simulink model "vco"  (R2019b)
settings: Solver=ode113  StartTime=0.0  StopTime=1e-6  RelTol=1e-3
values from neighbouring files (symbols this model uses):
  fs = fB*2    (= 10000000)    [vco_counter_m.m]    (also in vco_m.m = 1600000000)
  fvco = 1000e6    (= 1000000000)    [vco_counter_m.m]    (also in vco_m.m = 1600000000)
  ts = 1/fs    (= 1e-07)    [vco_counter_m.m]    (also in vco_m.m = 6.25e-10)
  tsys_res = 1e-11    [vco_counter_m.m]    (also in vco_m.m = 6.25e-10)
  tvco = 1/fvco    (= 6.25e-10)    [vco_m.m]
  vco_inverter_nums = 33    [vco_m.m]
libraries: simulink_extras x66
(part 1 of 2)
settings Model: Creator=benve  LastModifiedBy=benve

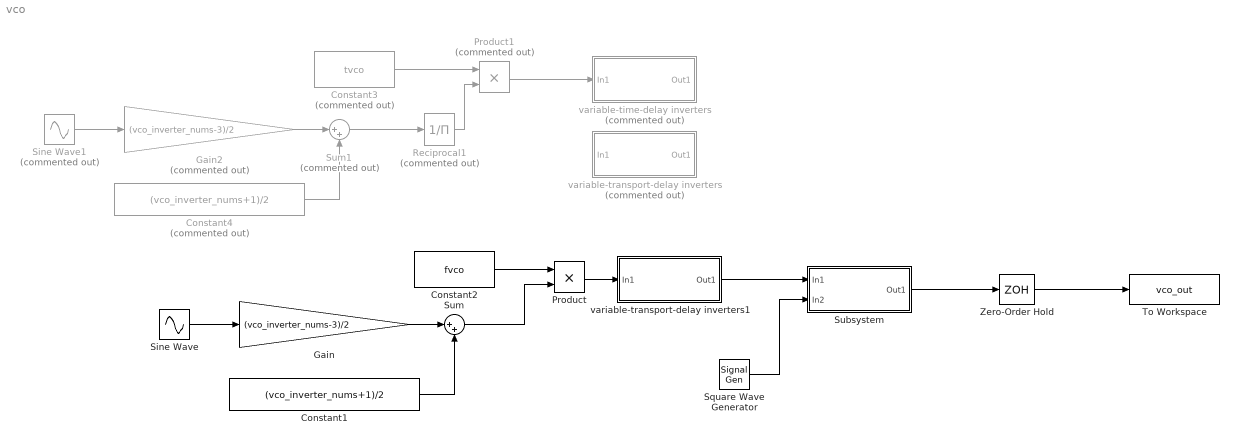
== system vco ==
  Constant1 : Constant  Value=(vco_inverter_nums+1)/2  SampleTime=tsys_res
  Constant2 : Constant  Value=fvco  SampleTime=tsys_res
  Constant3 : Constant  Commented=on  Value=tvco  SampleTime=tsys_res
  Constant4 : Constant  Commented=on  Value=(vco_inverter_nums+1)/2  SampleTime=tsys_res
  Gain : Gain  Gain=(vco_inverter_nums-3)/2
  Gain2 : Gain  Commented=on  Gain=(vco_inverter_nums-3)/2
  Product : Product
  Product1 : Product  Commented=on
  Reciprocal1 : Product  Commented=on  Inputs=/
  Sine Wave : Sin  Frequency=13e6*2*pi  SampleTime=ts
  Sine Wave1 : Sin  Commented=on  Frequency=13e6*2*pi  SampleTime=ts
  Square Wave Generator : SignalGenerator  WaveForm=square  Frequency=fs
  Subsystem : Subsystem
  Sum : Sum  Inputs=|++
  Sum1 : Sum  Commented=on  Inputs=|++
  To Workspace : ToWorkspace  VariableName=vco_out  SampleTime=-1
      settings: Save2DSignal=2-D array (concatenate along first dimension)
  Zero-Order Hold : ZeroOrderHold  SampleTime=ts
  variable-time-delay inverters : Subsystem  Commented=on  TreatAsAtomicUnit=on
      settings: RTWFcnNameOpts=Use subsystem name  RTWFileNameOpts=Use function name
  variable-transport-delay inverters : Subsystem  Commented=on  TreatAsAtomicUnit=on
      settings: RTWFcnNameOpts=Use subsystem name  RTWFileNameOpts=Use function name
  variable-transport-delay inverters1 : Subsystem  TreatAsAtomicUnit=on
      settings: RTWFcnNameOpts=Use subsystem name  RTWFileNameOpts=Use function name
  wires:
  Square Wave Generator/1 -> Subsystem/2(In2)
  Subsystem/1(Out1) -> Zero-Order Hold/1
  Zero-Order Hold/1 -> To Workspace/1
  variable-transport-delay inverters1/1(Out1) -> Subsystem/1(In1)
  Product/1 -> variable-transport-delay inverters1/1(In1)
  Reciprocal1/1 -> Product1/2
  Sine Wave1/1 -> Gain2/1
  Gain2/1 -> Sum1/1
  Constant3/1 -> Product1/1
  Constant4/1 -> Sum1/2
  Sum1/1 -> Reciprocal1/1
  Product1/1 -> variable-time-delay inverters/1(In1)
  Constant2/1 -> Product/1
  Sine Wave/1 -> Gain/1
  Gain/1 -> Sum/1
  Constant1/1 -> Sum/2
  Sum/1 -> Product/2

== system vco/Subsystem ==
  In1 : Inport
  In2 : Inport  Port=2
  "10 XORs " : Subsystem
  10 XORs 1 : Subsystem
  10 XORs 2 : Subsystem
  3 XORs : Subsystem
  Adder : Subsystem
  Bus Selector : BusSelector  OutputSignals=signal1,signal2,signal3,signal4
  stage1 - 10registers : Subsystem
  stage1 - 10registers1 : Subsystem
  stage1 - 10registers2 : Subsystem
  stage1 - 3registers : Subsystem
  stage2 - 10registers1 : Subsystem
  stage2 - 10registers2 : Subsystem
  stage2 - 10registers3 : Subsystem
  stage2 - 3registers : Subsystem
  Out1 : Outport
  wires:
  "10 XORs "/1(Out2) -> Adder/1(In1)
  stage2 - 10registers3/1(Out1) -> "10 XORs "/2(In3)
  Adder/1(Out1) -> Out1/1
  Bus Selector/4 -> stage1 - 3registers/1(In1)  "<signal4>"
  stage2 - 10registers1/1(Out1) -> 10 XORs 1/2(In3)
  stage2 - 10registers2/1(Out1) -> 10 XORs 2/2(In3)
  10 XORs 1/1(Out2) -> Adder/2(In2)
  Bus Selector/3 -> stage1 - 10registers2/1(In1)  "<signal3>"
  stage1 - 10registers1/1(Out1) -> 10 XORs 1/1(In2), stage2 - 10registers1/1(In1)
  10 XORs 2/1(Out2) -> Adder/3(In3)
  stage1 - 3registers/1(Out1) -> 3 XORs/1(In1), stage2 - 3registers/1(In1)
  In2/1 -> stage2 - 3registers/2(In2), stage2 - 10registers3/2(In2), stage2 - 10registers1/2(In2), stage2 - 10registers2/2(In2), stage1 - 3registers/2(In2), stage1 - 10registers2/2(In2), stage1 - 10registers/2(In2), stage1 - 10registers1/2(In2)  "SAMP_CLK"
  In1/1 -> Bus Selector/1
  stage1 - 10registers2/1(Out1) -> 10 XORs 2/1(In2), stage2 - 10registers2/1(In1)
  3 XORs/1(Out1) -> Adder/4(In4)
  stage2 - 3registers/1(Out1) -> 3 XORs/2(In2)
  Bus Selector/2 -> stage1 - 10registers1/1(In1)  "<signal2>"
  stage1 - 10registers/1(Out1) -> "10 XORs "/1(In2), stage2 - 10registers3/1(In1)
  Bus Selector/1 -> stage1 - 10registers/1(In1)  "<signal1>"

== system vco/variable-time-delay inverters ==
  In1 : Inport
  " 3 inverters" : Subsystem
  10 inverters : Subsystem
  10 inverters1 : Subsystem
  10 inverters2 : Subsystem
  Bus Creator : BusCreator  Inputs=4
  Out1 : Outport
  wires:
  Bus Creator/1 -> Out1/1
  10 inverters/1(Out2) -> 10 inverters1/1(In1)
  10 inverters1/1(Out2) -> 10 inverters2/1(In1)
  10 inverters2/1(Out2) -> " 3 inverters"/1(In1)
  10 inverters/2(Out1) -> Bus Creator/1
  10 inverters1/2(Out1) -> Bus Creator/2
  10 inverters2/2(Out1) -> Bus Creator/3
  " 3 inverters"/1(Out2) -> 10 inverters/1(In1)
  In1/1 -> 10 inverters1/2(In2), 10 inverters2/2(In2), " 3 inverters"/2(In2), 10 inverters/2(In2)  "delay"
  " 3 inverters"/2(Out1) -> Bus Creator/4

== system vco/variable-transport-delay inverters ==
  In1 : Inport
  " 3 inverters" : Subsystem
  10 inverters : Subsystem
  10 inverters1 : Subsystem
  10 inverters2 : Subsystem
  Bus Creator : BusCreator  Inputs=4
  Out1 : Outport
  wires:
  Bus Creator/1 -> Out1/1
  10 inverters/1(Out2) -> 10 inverters1/1(In1)
  10 inverters1/1(Out2) -> 10 inverters2/1(In1)
  10 inverters2/1(Out2) -> " 3 inverters"/1(In1)
  10 inverters/2(Out1) -> Bus Creator/1
  10 inverters1/2(Out1) -> Bus Creator/2
  10 inverters2/2(Out1) -> Bus Creator/3
  " 3 inverters"/1(Out2) -> 10 inverters/1(In1)
  In1/1 -> 10 inverters1/2(In2), 10 inverters2/2(In2), " 3 inverters"/2(In2), 10 inverters/2(In2)  "delay"
  " 3 inverters"/2(Out1) -> Bus Creator/4

== system vco/variable-transport-delay inverters1 ==
  In1 : Inport
  10 inverters : Subsystem
  10 inverters1 : Subsystem
  10 inverters2 : Subsystem
  3 inverters : Subsystem
  Bus Creator : BusCreator  Inputs=4
  Out1 : Outport
  wires:
  Bus Creator/1 -> Out1/1
  10 inverters1/1(Out2) -> 10 inverters2/1(In1)
  10 inverters2/1(Out2) -> 3 inverters/1(In1)
  10 inverters1/2(Out1) -> Bus Creator/2
  10 inverters2/2(Out1) -> Bus Creator/3
  In1/1 -> 10 inverters/2(In2), 10 inverters1/2(In2), 10 inverters2/2(In2), 3 inverters/2(In2)  "delay"
  10 inverters/1(Out2) -> 10 inverters1/1(In1)
  10 inverters/2(Out1) -> Bus Creator/1
  3 inverters/1(Out2) -> 10 inverters/1(In1)
  3 inverters/2(Out1) -> Bus Creator/4

== system vco/Subsystem/10 XORs  ==
  In2 : Inport
  In3 : Inport  Port=2
  Bus Creator : BusCreator  Inputs=2
  Bus Creator1 : BusCreator  Inputs=10
  Bus Selector2 : BusSelector  OutputSignals=signal1.signal1,signal2.signal1,signal1.signal2,signal2.signal2,signal1.signal3,signal2.signal3,signal1.signal4,signal2.signal4,signal1.signal5,signal2.signal5,signal1.signal6,signal2.signal6,signal1.signal7,signal2.signal7,signal1.signal8,signal2.signal8,signal1.signal9,signal2.signal9,signal1.signal10,signal2.signal10
  XOR{,1..9} (10 alike) : Logic  Operator=XOR  IconShape=distinctive  AllPortsSameDT=off  OutDataTypeStr=boolean
  Out2 : Outport
  wires:
  XOR2/1 -> Bus Creator1/3
  XOR/1 -> Bus Creator1/1
  Bus Selector2/19 -> XOR9/1  "<signal10>"
  XOR7/1 -> Bus Creator1/8
  Bus Selector2/13 -> XOR6/1  "<signal7>"
  XOR8/1 -> Bus Creator1/9
  XOR9/1 -> Bus Creator1/10
  Bus Selector2/16 -> XOR7/2  "<signal8>"
  Bus Selector2/5 -> XOR2/1  "<signal3>"
  Bus Selector2/17 -> XOR8/1  "<signal9>"
  Bus Creator1/1 -> Out2/1
  Bus Selector2/9 -> XOR4/1  "<signal5>"
  XOR5/1 -> Bus Creator1/6
  XOR6/1 -> Bus Creator1/7
  Bus Selector2/18 -> XOR8/2  "<signal9>"
  XOR1/1 -> Bus Creator1/2
  Bus Selector2/12 -> XOR5/2  "<signal6>"
  Bus Selector2/3 -> XOR1/1  "<signal2>"
  Bus Selector2/4 -> XOR1/2  "<signal2>"
  Bus Selector2/15 -> XOR7/1  "<signal8>"
  Bus Selector2/11 -> XOR5/1  "<signal6>"
  In3/1 -> Bus Creator/2
  Bus Selector2/8 -> XOR3/2  "<signal4>"
  Bus Selector2/6 -> XOR2/2  "<signal3>"
  Bus Selector2/14 -> XOR6/2  "<signal7>"
  Bus Creator/1 -> Bus Selector2/1
  XOR4/1 -> Bus Creator1/5
  Bus Selector2/2 -> XOR/2  "<signal1>"
  Bus Selector2/10 -> XOR4/2  "<signal5>"
  Bus Selector2/7 -> XOR3/1  "<signal4>"
  Bus Selector2/1 -> XOR/1  "<signal1>"
  Bus Selector2/20 -> XOR9/2  "<signal10>"
  In2/1 -> Bus Creator/1
  XOR3/1 -> Bus Creator1/4

== system vco/Subsystem/10 XORs 1 ==
  In2 : Inport
  In3 : Inport  Port=2
  Bus Creator : BusCreator  Inputs=2
  Bus Creator1 : BusCreator  Inputs=10
  Bus Selector2 : BusSelector  OutputSignals=signal1.signal1,signal2.signal1,signal1.signal2,signal2.signal2,signal1.signal3,signal2.signal3,signal1.signal4,signal2.signal4,signal1.signal5,signal2.signal5,signal1.signal6,signal2.signal6,signal1.signal7,signal2.signal7,signal1.signal8,signal2.signal8,signal1.signal9,signal2.signal9,signal1.signal10,signal2.signal10
  XOR{,1..9} (10 alike) : Logic  Operator=XOR  IconShape=distinctive  AllPortsSameDT=off  OutDataTypeStr=boolean
  Out2 : Outport
  wires:
  XOR2/1 -> Bus Creator1/3
  XOR/1 -> Bus Creator1/1
  Bus Selector2/19 -> XOR9/1  "<signal10>"
  XOR7/1 -> Bus Creator1/8
  Bus Selector2/13 -> XOR6/1  "<signal7>"
  XOR8/1 -> Bus Creator1/9
  XOR9/1 -> Bus Creator1/10
  Bus Selector2/16 -> XOR7/2  "<signal8>"
  Bus Selector2/5 -> XOR2/1  "<signal3>"
  Bus Selector2/17 -> XOR8/1  "<signal9>"
  Bus Creator1/1 -> Out2/1
  Bus Selector2/9 -> XOR4/1  "<signal5>"
  XOR5/1 -> Bus Creator1/6
  XOR6/1 -> Bus Creator1/7
  Bus Selector2/18 -> XOR8/2  "<signal9>"
  XOR1/1 -> Bus Creator1/2
  Bus Selector2/12 -> XOR5/2  "<signal6>"
  Bus Selector2/3 -> XOR1/1  "<signal2>"
  Bus Selector2/4 -> XOR1/2  "<signal2>"
  Bus Selector2/15 -> XOR7/1  "<signal8>"
  Bus Selector2/11 -> XOR5/1  "<signal6>"
  In3/1 -> Bus Creator/2
  Bus Selector2/8 -> XOR3/2  "<signal4>"
  Bus Selector2/6 -> XOR2/2  "<signal3>"
  Bus Selector2/14 -> XOR6/2  "<signal7>"
  Bus Creator/1 -> Bus Selector2/1
  XOR4/1 -> Bus Creator1/5
  Bus Selector2/2 -> XOR/2  "<signal1>"
  Bus Selector2/10 -> XOR4/2  "<signal5>"
  Bus Selector2/7 -> XOR3/1  "<signal4>"
  Bus Selector2/1 -> XOR/1  "<signal1>"
  Bus Selector2/20 -> XOR9/2  "<signal10>"
  In2/1 -> Bus Creator/1
  XOR3/1 -> Bus Creator1/4

== system vco/Subsystem/10 XORs 2 ==
  In2 : Inport
  In3 : Inport  Port=2
  Bus Creator : BusCreator  Inputs=2
  Bus Creator1 : BusCreator  Inputs=10
  Bus Selector2 : BusSelector  OutputSignals=signal1.signal1,signal2.signal1,signal1.signal2,signal2.signal2,signal1.signal3,signal2.signal3,signal1.signal4,signal2.signal4,signal1.signal5,signal2.signal5,signal1.signal6,signal2.signal6,signal1.signal7,signal2.signal7,signal1.signal8,signal2.signal8,signal1.signal9,signal2.signal9,signal1.signal10,signal2.signal10
  XOR{,1..9} (10 alike) : Logic  Operator=XOR  IconShape=distinctive  AllPortsSameDT=off  OutDataTypeStr=boolean
  Out2 : Outport
  wires:
  XOR2/1 -> Bus Creator1/3
  XOR/1 -> Bus Creator1/1
  Bus Selector2/19 -> XOR9/1  "<signal10>"
  XOR7/1 -> Bus Creator1/8
  Bus Selector2/13 -> XOR6/1  "<signal7>"
  XOR8/1 -> Bus Creator1/9
  XOR9/1 -> Bus Creator1/10
  Bus Selector2/16 -> XOR7/2  "<signal8>"
  Bus Selector2/5 -> XOR2/1  "<signal3>"
  Bus Selector2/17 -> XOR8/1  "<signal9>"
  Bus Creator1/1 -> Out2/1
  Bus Selector2/9 -> XOR4/1  "<signal5>"
  XOR5/1 -> Bus Creator1/6
  XOR6/1 -> Bus Creator1/7
  Bus Selector2/18 -> XOR8/2  "<signal9>"
  XOR1/1 -> Bus Creator1/2
  Bus Selector2/12 -> XOR5/2  "<signal6>"
  Bus Selector2/3 -> XOR1/1  "<signal2>"
  Bus Selector2/4 -> XOR1/2  "<signal2>"
  Bus Selector2/15 -> XOR7/1  "<signal8>"
  Bus Selector2/11 -> XOR5/1  "<signal6>"
  In3/1 -> Bus Creator/2
  Bus Selector2/8 -> XOR3/2  "<signal4>"
  Bus Selector2/6 -> XOR2/2  "<signal3>"
  Bus Selector2/14 -> XOR6/2  "<signal7>"
  Bus Creator/1 -> Bus Selector2/1
  XOR4/1 -> Bus Creator1/5
  Bus Selector2/2 -> XOR/2  "<signal1>"
  Bus Selector2/10 -> XOR4/2  "<signal5>"
  Bus Selector2/7 -> XOR3/1  "<signal4>"
  Bus Selector2/1 -> XOR/1  "<signal1>"
  Bus Selector2/20 -> XOR9/2  "<signal10>"
  In2/1 -> Bus Creator/1
  XOR3/1 -> Bus Creator1/4

== system vco/Subsystem/3 XORs ==
  In1 : Inport
  In2 : Inport  Port=2
  Bus Creator : BusCreator  Inputs=2
  Bus Creator1 : BusCreator  Inputs=3
  Bus Selector2 : BusSelector  OutputSignals=signal1.signal1,signal2.signal1,signal1.signal2,signal2.signal2,signal1.signal3,signal2.signal3
  XOR : Logic  Operator=XOR  IconShape=distinctive  AllPortsSameDT=off  OutDataTypeStr=boolean
  XOR1 : Logic  Operator=XOR  IconShape=distinctive  AllPortsSameDT=off  OutDataTypeStr=boolean
  XOR2 : Logic  Operator=XOR  IconShape=distinctive  AllPortsSameDT=off  OutDataTypeStr=boolean
  Out1 : Outport
  wires:
  XOR2/1 -> Bus Creator1/3
  XOR1/1 -> Bus Creator1/2
  XOR/1 -> Bus Creator1/1
  Bus Creator1/1 -> Out1/1
  Bus Selector2/6 -> XOR2/2  "<signal3>"
  Bus Selector2/4 -> XOR1/2  "<signal2>"
  In2/1 -> Bus Creator/2
  Bus Selector2/5 -> XOR2/1  "<signal3>"
  Bus Selector2/1 -> XOR/1  "<signal1>"
  Bus Selector2/3 -> XOR1/1  "<signal2>"
  Bus Creator/1 -> Bus Selector2/1
  Bus Selector2/2 -> XOR/2  "<signal1>"
  In1/1 -> Bus Creator/1

== system vco/Subsystem/Adder ==
  In1 : Inport
  In2 : Inport  Port=2
  In3 : Inport  Port=3
  In4 : Inport  Port=4
  Add : Sum  Inputs=++++++++++
  Add1 : Sum  Inputs=++++++++++
  Add2 : Sum  Inputs=++++++++++
  Add3 : Sum  Inputs=+++
  Add4 : Sum  Inputs=++++
  Bus Selector : BusSelector  OutputSignals=signal1,signal2,signal3,signal4,signal5,signal6,signal7,signal8,signal9,signal10
  Bus Selector1 : BusSelector  OutputSignals=signal1,signal2,signal3,signal4,signal5,signal6,signal7,signal8,signal9,signal10
  Bus Selector2 : BusSelector  OutputSignals=signal1,signal2,signal3,signal4,signal5,signal6,signal7,signal8,signal9,signal10
  Bus Selector3 : BusSelector  OutputSignals=signal1,signal2,signal3
  Out1 : Outport
  wires:
  In1/1 -> Bus Selector/1
  Bus Selector/1 -> Add/1  "<signal1>"
  Bus Selector/2 -> Add/2  "<signal2>"
  Bus Selector/3 -> Add/3  "<signal3>"
  Bus Selector/4 -> Add/4  "<signal4>"
  Bus Selector/5 -> Add/5  "<signal5>"
  Bus Selector/6 -> Add/6  "<signal6>"
  Bus Selector/7 -> Add/7  "<signal7>"
  Bus Selector/8 -> Add/8  "<signal8>"
  Bus Selector/9 -> Add/9  "<signal9>"
  Bus Selector/10 -> Add/10  "<signal10>"
  Bus Selector1/10 -> Add1/10  "<signal10>"
  In2/1 -> Bus Selector1/1
  Bus Selector1/4 -> Add1/4  "<signal4>"
  Bus Selector1/2 -> Add1/2  "<signal2>"
  Bus Selector1/6 -> Add1/6  "<signal6>"
  Bus Selector1/3 -> Add1/3  "<signal3>"
  Bus Selector1/5 -> Add1/5  "<signal5>"
  Bus Selector1/9 -> Add1/9  "<signal9>"
  Bus Selector1/7 -> Add1/7  "<signal7>"
  Bus Selector1/1 -> Add1/1  "<signal1>"
  Bus Selector1/8 -> Add1/8  "<signal8>"
  Bus Selector2/10 -> Add2/10  "<signal10>"
  In3/1 -> Bus Selector2/1
  Bus Selector3/1 -> Add3/1  "<signal1>"
  In4/1 -> Bus Selector3/1
  Bus Selector3/2 -> Add3/2  "<signal2>"
  Bus Selector2/4 -> Add2/4  "<signal4>"
  Bus Selector2/2 -> Add2/2  "<signal2>"
  Bus Selector2/6 -> Add2/6  "<signal6>"
  Bus Selector2/3 -> Add2/3  "<signal3>"
  Bus Selector2/5 -> Add2/5  "<signal5>"
  Bus Selector2/9 -> Add2/9  "<signal9>"
  Bus Selector2/7 -> Add2/7  "<signal7>"
  Bus Selector2/1 -> Add2/1  "<signal1>"
  Bus Selector2/8 -> Add2/8  "<signal8>"
  Bus Selector3/3 -> Add3/3  "<signal3>"
  Add3/1 -> Add4/4
  Add2/1 -> Add4/3
  Add1/1 -> Add4/2
  Add/1 -> Add4/1
  Add4/1 -> Out1/1

== system vco/Subsystem/stage1 - 10registers ==
  In1 : Inport
  In2 : Inport  Port=2
  Bus Creator : BusCreator  Inputs=10
  Bus Selector : BusSelector  OutputSignals=signal10,signal9,signal8,signal7,signal6,signal5,signal4,signal3,signal2,signal1
  Constant1 : Constant  SampleTime=1e-11
  D Flip-Flop{,1..9} (10 alike) : simulink_extras/Flip Flops/D Flip-Flop
      settings: SourceProductName=Simulink
  Out1 : Outport
  wires:
  Constant1/1 -> D Flip-Flop9/3, D Flip-Flop8/3, D Flip-Flop7/3, D Flip-Flop6/3, D Flip-Flop5/3, D Flip-Flop4/3, D Flip-Flop3/3, D Flip-Flop2/3, D Flip-Flop1/3, D Flip-Flop/3
  In2/1 -> D Flip-Flop9/2, D Flip-Flop8/2, D Flip-Flop7/2, D Flip-Flop6/2, D Flip-Flop5/2, D Flip-Flop4/2, D Flip-Flop3/2, D Flip-Flop2/2, D Flip-Flop1/2, D Flip-Flop/2  "CLK"
  Bus Selector/10 -> D Flip-Flop/1  "<signal1>"
  Bus Selector/9 -> D Flip-Flop1/1  "<signal2>"
  Bus Selector/8 -> D Flip-Flop2/1  "<signal3>"
  Bus Selector/7 -> D Flip-Flop3/1  "<signal4>"
  Bus Selector/6 -> D Flip-Flop4/1  "<signal5>"
  Bus Selector/5 -> D Flip-Flop5/1  "<signal6>"
  Bus Selector/3 -> D Flip-Flop7/1  "<signal8>"
  Bus Selector/4 -> D Flip-Flop6/1  "<signal7>"
  Bus Selector/2 -> D Flip-Flop8/1  "<signal9>"
  Bus Selector/1 -> D Flip-Flop9/1  "<signal10>"
  D Flip-Flop/1 -> Bus Creator/1
  D Flip-Flop1/1 -> Bus Creator/2
  D Flip-Flop2/1 -> Bus Creator/3
  D Flip-Flop3/1 -> Bus Creator/4
  D Flip-Flop4/1 -> Bus Creator/5
  D Flip-Flop5/1 -> Bus Creator/6
  D Flip-Flop6/1 -> Bus Creator/7
  D Flip-Flop7/1 -> Bus Creator/8
  D Flip-Flop8/1 -> Bus Creator/9
  D Flip-Flop9/1 -> Bus Creator/10
  Bus Creator/1 -> Out1/1
  In1/1 -> Bus Selector/1

== system vco/Subsystem/stage1 - 10registers1 ==
  In1 : Inport
  In2 : Inport  Port=2
  Bus Creator : BusCreator  Inputs=10
  Bus Selector : BusSelector  OutputSignals=signal10,signal9,signal8,signal7,signal6,signal5,signal4,signal3,signal2,signal1
  Constant1 : Constant  SampleTime=1e-11
  D Flip-Flop{,1..9} (10 alike) : simulink_extras/Flip Flops/D Flip-Flop
      settings: SourceProductName=Simulink
  Out1 : Outport
  wires:
  Constant1/1 -> D Flip-Flop9/3, D Flip-Flop8/3, D Flip-Flop7/3, D Flip-Flop6/3, D Flip-Flop5/3, D Flip-Flop4/3, D Flip-Flop3/3, D Flip-Flop2/3, D Flip-Flop1/3, D Flip-Flop/3
  In2/1 -> D Flip-Flop9/2, D Flip-Flop8/2, D Flip-Flop7/2, D Flip-Flop6/2, D Flip-Flop5/2, D Flip-Flop4/2, D Flip-Flop3/2, D Flip-Flop2/2, D Flip-Flop1/2, D Flip-Flop/2  "CLK"
  Bus Selector/10 -> D Flip-Flop/1  "<signal1>"
  Bus Selector/9 -> D Flip-Flop1/1  "<signal2>"
  Bus Selector/8 -> D Flip-Flop2/1  "<signal3>"
  Bus Selector/7 -> D Flip-Flop3/1  "<signal4>"
  Bus Selector/6 -> D Flip-Flop4/1  "<signal5>"
  Bus Selector/5 -> D Flip-Flop5/1  "<signal6>"
  Bus Selector/3 -> D Flip-Flop7/1  "<signal8>"
  Bus Selector/4 -> D Flip-Flop6/1  "<signal7>"
  Bus Selector/2 -> D Flip-Flop8/1  "<signal9>"
  Bus Selector/1 -> D Flip-Flop9/1  "<signal10>"
  D Flip-Flop/1 -> Bus Creator/1
  D Flip-Flop1/1 -> Bus Creator/2
  D Flip-Flop2/1 -> Bus Creator/3
  D Flip-Flop3/1 -> Bus Creator/4
  D Flip-Flop4/1 -> Bus Creator/5
  D Flip-Flop5/1 -> Bus Creator/6
  D Flip-Flop6/1 -> Bus Creator/7
  D Flip-Flop7/1 -> Bus Creator/8
  D Flip-Flop8/1 -> Bus Creator/9
  D Flip-Flop9/1 -> Bus Creator/10
  Bus Creator/1 -> Out1/1
  In1/1 -> Bus Selector/1

== system vco/Subsystem/stage1 - 10registers2 ==
  In1 : Inport
  In2 : Inport  Port=2
  Bus Creator : BusCreator  Inputs=10
  Bus Selector : BusSelector  OutputSignals=signal10,signal9,signal8,signal7,signal6,signal5,signal4,signal3,signal2,signal1
  Constant1 : Constant  SampleTime=1e-11
  D Flip-Flop{,1..9} (10 alike) : simulink_extras/Flip Flops/D Flip-Flop
      settings: SourceProductName=Simulink
  Out1 : Outport
  wires:
  Constant1/1 -> D Flip-Flop9/3, D Flip-Flop8/3, D Flip-Flop7/3, D Flip-Flop6/3, D Flip-Flop5/3, D Flip-Flop4/3, D Flip-Flop3/3, D Flip-Flop2/3, D Flip-Flop1/3, D Flip-Flop/3
  In2/1 -> D Flip-Flop9/2, D Flip-Flop8/2, D Flip-Flop7/2, D Flip-Flop6/2, D Flip-Flop5/2, D Flip-Flop4/2, D Flip-Flop3/2, D Flip-Flop2/2, D Flip-Flop1/2, D Flip-Flop/2  "CLK"
  Bus Selector/10 -> D Flip-Flop/1  "<signal1>"
  Bus Selector/9 -> D Flip-Flop1/1  "<signal2>"
  Bus Selector/8 -> D Flip-Flop2/1  "<signal3>"
  Bus Selector/7 -> D Flip-Flop3/1  "<signal4>"
  Bus Selector/6 -> D Flip-Flop4/1  "<signal5>"
  Bus Selector/5 -> D Flip-Flop5/1  "<signal6>"
  Bus Selector/3 -> D Flip-Flop7/1  "<signal8>"
  Bus Selector/4 -> D Flip-Flop6/1  "<signal7>"
  Bus Selector/2 -> D Flip-Flop8/1  "<signal9>"
  Bus Selector/1 -> D Flip-Flop9/1  "<signal10>"
  D Flip-Flop/1 -> Bus Creator/1
  D Flip-Flop1/1 -> Bus Creator/2
  D Flip-Flop2/1 -> Bus Creator/3
  D Flip-Flop3/1 -> Bus Creator/4
  D Flip-Flop4/1 -> Bus Creator/5
  D Flip-Flop5/1 -> Bus Creator/6
  D Flip-Flop6/1 -> Bus Creator/7
  D Flip-Flop7/1 -> Bus Creator/8
  D Flip-Flop8/1 -> Bus Creator/9
  D Flip-Flop9/1 -> Bus Creator/10
  Bus Creator/1 -> Out1/1
  In1/1 -> Bus Selector/1

== system vco/Subsystem/stage1 - 3registers ==
  In1 : Inport
  In2 : Inport  Port=2
  Bus Creator : BusCreator  Inputs=3
  Bus Selector : BusSelector  OutputSignals=signal3,signal2,signal1
  Constant1 : Constant  SampleTime=1e-11
  D Flip-Flop : simulink_extras/Flip Flops/D Flip-Flop
      settings: SourceProductName=Simulink
  D Flip-Flop1 : simulink_extras/Flip Flops/D Flip-Flop
      settings: SourceProductName=Simulink
  D Flip-Flop2 : simulink_extras/Flip Flops/D Flip-Flop
      settings: SourceProductName=Simulink
  Out1 : Outport
  wires:
  Constant1/1 -> D Flip-Flop2/3, D Flip-Flop1/3, D Flip-Flop/3
  In2/1 -> D Flip-Flop2/2, D Flip-Flop1/2, D Flip-Flop/2  "CLK"
  Bus Selector/3 -> D Flip-Flop/1  "<signal1>"
  Bus Selector/2 -> D Flip-Flop1/1  "<signal2>"
  Bus Selector/1 -> D Flip-Flop2/1  "<signal3>"
  D Flip-Flop/1 -> Bus Creator/1
  D Flip-Flop1/1 -> Bus Creator/2
  D Flip-Flop2/1 -> Bus Creator/3
  Bus Creator/1 -> Out1/1
  In1/1 -> Bus Selector/1

== system vco/Subsystem/stage2 - 10registers1 ==
  In1 : Inport
  In2 : Inport  Port=2
  Bus Creator : BusCreator  Inputs=10
  Bus Selector : BusSelector  OutputSignals=signal10,signal9,signal8,signal7,signal6,signal5,signal4,signal3,signal2,signal1
  Constant1 : Constant  SampleTime=1e-11
  D Flip-Flop{,1..9} (10 alike) : simulink_extras/Flip Flops/D Flip-Flop
      settings: SourceProductName=Simulink
  Out1 : Outport
  wires:
  Constant1/1 -> D Flip-Flop9/3, D Flip-Flop8/3, D Flip-Flop7/3, D Flip-Flop6/3, D Flip-Flop5/3, D Flip-Flop4/3, D Flip-Flop3/3, D Flip-Flop2/3, D Flip-Flop1/3, D Flip-Flop/3
  In2/1 -> D Flip-Flop9/2, D Flip-Flop8/2, D Flip-Flop7/2, D Flip-Flop6/2, D Flip-Flop5/2, D Flip-Flop4/2, D Flip-Flop3/2, D Flip-Flop2/2, D Flip-Flop1/2, D Flip-Flop/2  "CLK"
  Bus Selector/10 -> D Flip-Flop/1  "<signal1>"
  Bus Selector/9 -> D Flip-Flop1/1  "<signal2>"
  Bus Selector/8 -> D Flip-Flop2/1  "<signal3>"
  Bus Selector/7 -> D Flip-Flop3/1  "<signal4>"
  Bus Selector/6 -> D Flip-Flop4/1  "<signal5>"
  Bus Selector/5 -> D Flip-Flop5/1  "<signal6>"
  Bus Selector/3 -> D Flip-Flop7/1  "<signal8>"
  Bus Selector/4 -> D Flip-Flop6/1  "<signal7>"
  Bus Selector/2 -> D Flip-Flop8/1  "<signal9>"
  Bus Selector/1 -> D Flip-Flop9/1  "<signal10>"
  D Flip-Flop/1 -> Bus Creator/1
  D Flip-Flop1/1 -> Bus Creator/2
  D Flip-Flop2/1 -> Bus Creator/3
  D Flip-Flop3/1 -> Bus Creator/4
  D Flip-Flop4/1 -> Bus Creator/5
  D Flip-Flop5/1 -> Bus Creator/6
  D Flip-Flop6/1 -> Bus Creator/7
  D Flip-Flop7/1 -> Bus Creator/8
  D Flip-Flop8/1 -> Bus Creator/9
  D Flip-Flop9/1 -> Bus Creator/10
  Bus Creator/1 -> Out1/1
  In1/1 -> Bus Selector/1

== system vco/Subsystem/stage2 - 10registers2 ==
  In1 : Inport
  In2 : Inport  Port=2
  Bus Creator : BusCreator  Inputs=10
  Bus Selector : BusSelector  OutputSignals=signal10,signal9,signal8,signal7,signal6,signal5,signal4,signal3,signal2,signal1
  Constant1 : Constant  SampleTime=1e-11
  D Flip-Flop{,1..9} (10 alike) : simulink_extras/Flip Flops/D Flip-Flop
      settings: SourceProductName=Simulink
  Out1 : Outport
  wires:
  Constant1/1 -> D Flip-Flop9/3, D Flip-Flop8/3, D Flip-Flop7/3, D Flip-Flop6/3, D Flip-Flop5/3, D Flip-Flop4/3, D Flip-Flop3/3, D Flip-Flop2/3, D Flip-Flop1/3, D Flip-Flop/3
  In2/1 -> D Flip-Flop9/2, D Flip-Flop8/2, D Flip-Flop7/2, D Flip-Flop6/2, D Flip-Flop5/2, D Flip-Flop4/2, D Flip-Flop3/2, D Flip-Flop2/2, D Flip-Flop1/2, D Flip-Flop/2  "CLK"
  Bus Selector/10 -> D Flip-Flop/1  "<signal1>"
  Bus Selector/9 -> D Flip-Flop1/1  "<signal2>"
  Bus Selector/8 -> D Flip-Flop2/1  "<signal3>"
  Bus Selector/7 -> D Flip-Flop3/1  "<signal4>"
  Bus Selector/6 -> D Flip-Flop4/1  "<signal5>"
  Bus Selector/5 -> D Flip-Flop5/1  "<signal6>"
  Bus Selector/3 -> D Flip-Flop7/1  "<signal8>"
  Bus Selector/4 -> D Flip-Flop6/1  "<signal7>"
  Bus Selector/2 -> D Flip-Flop8/1  "<signal9>"
  Bus Selector/1 -> D Flip-Flop9/1  "<signal10>"
  D Flip-Flop/1 -> Bus Creator/1
  D Flip-Flop1/1 -> Bus Creator/2
  D Flip-Flop2/1 -> Bus Creator/3
  D Flip-Flop3/1 -> Bus Creator/4
  D Flip-Flop4/1 -> Bus Creator/5
  D Flip-Flop5/1 -> Bus Creator/6
  D Flip-Flop6/1 -> Bus Creator/7
  D Flip-Flop7/1 -> Bus Creator/8
  D Flip-Flop8/1 -> Bus Creator/9
  D Flip-Flop9/1 -> Bus Creator/10
  Bus Creator/1 -> Out1/1
  In1/1 -> Bus Selector/1

== system vco/Subsystem/stage2 - 10registers3 ==
  In1 : Inport
  In2 : Inport  Port=2
  Bus Creator : BusCreator  Inputs=10
  Bus Selector : BusSelector  OutputSignals=signal10,signal9,signal8,signal7,signal6,signal5,signal4,signal3,signal2,signal1
  Constant1 : Constant  SampleTime=1e-11
  D Flip-Flop{,1..9} (10 alike) : simulink_extras/Flip Flops/D Flip-Flop
      settings: SourceProductName=Simulink
  Out1 : Outport
  wires:
  Constant1/1 -> D Flip-Flop9/3, D Flip-Flop8/3, D Flip-Flop7/3, D Flip-Flop6/3, D Flip-Flop5/3, D Flip-Flop4/3, D Flip-Flop3/3, D Flip-Flop2/3, D Flip-Flop1/3, D Flip-Flop/3
  In2/1 -> D Flip-Flop9/2, D Flip-Flop8/2, D Flip-Flop7/2, D Flip-Flop6/2, D Flip-Flop5/2, D Flip-Flop4/2, D Flip-Flop3/2, D Flip-Flop2/2, D Flip-Flop1/2, D Flip-Flop/2  "CLK"
  Bus Selector/10 -> D Flip-Flop/1  "<signal1>"
  Bus Selector/9 -> D Flip-Flop1/1  "<signal2>"
  Bus Selector/8 -> D Flip-Flop2/1  "<signal3>"
  Bus Selector/7 -> D Flip-Flop3/1  "<signal4>"
  Bus Selector/6 -> D Flip-Flop4/1  "<signal5>"
  Bus Selector/5 -> D Flip-Flop5/1  "<signal6>"
  Bus Selector/3 -> D Flip-Flop7/1  "<signal8>"
  Bus Selector/4 -> D Flip-Flop6/1  "<signal7>"
  Bus Selector/2 -> D Flip-Flop8/1  "<signal9>"
  Bus Selector/1 -> D Flip-Flop9/1  "<signal10>"
  D Flip-Flop/1 -> Bus Creator/1
  D Flip-Flop1/1 -> Bus Creator/2
  D Flip-Flop2/1 -> Bus Creator/3
  D Flip-Flop3/1 -> Bus Creator/4
  D Flip-Flop4/1 -> Bus Creator/5
  D Flip-Flop5/1 -> Bus Creator/6
  D Flip-Flop6/1 -> Bus Creator/7
  D Flip-Flop7/1 -> Bus Creator/8
  D Flip-Flop8/1 -> Bus Creator/9
  D Flip-Flop9/1 -> Bus Creator/10
  Bus Creator/1 -> Out1/1
  In1/1 -> Bus Selector/1

== system vco/Subsystem/stage2 - 3registers ==
  In1 : Inport
  In2 : Inport  Port=2
  Bus Creator : BusCreator  Inputs=3
  Bus Selector : BusSelector  OutputSignals=signal3,signal2,signal1
  Constant1 : Constant  SampleTime=1e-11
  D Flip-Flop : simulink_extras/Flip Flops/D Flip-Flop
      settings: SourceProductName=Simulink
  D Flip-Flop1 : simulink_extras/Flip Flops/D Flip-Flop
      settings: SourceProductName=Simulink
  D Flip-Flop2 : simulink_extras/Flip Flops/D Flip-Flop
      settings: SourceProductName=Simulink
  Out1 : Outport
  wires:
  Constant1/1 -> D Flip-Flop2/3, D Flip-Flop1/3, D Flip-Flop/3
  In2/1 -> D Flip-Flop2/2, D Flip-Flop1/2, D Flip-Flop/2  "CLK"
  Bus Selector/3 -> D Flip-Flop/1  "<signal1>"
  Bus Selector/2 -> D Flip-Flop1/1  "<signal2>"
  Bus Selector/1 -> D Flip-Flop2/1  "<signal3>"
  D Flip-Flop/1 -> Bus Creator/1
  D Flip-Flop1/1 -> Bus Creator/2
  D Flip-Flop2/1 -> Bus Creator/3
  Bus Creator/1 -> Out1/1
  In1/1 -> Bus Selector/1

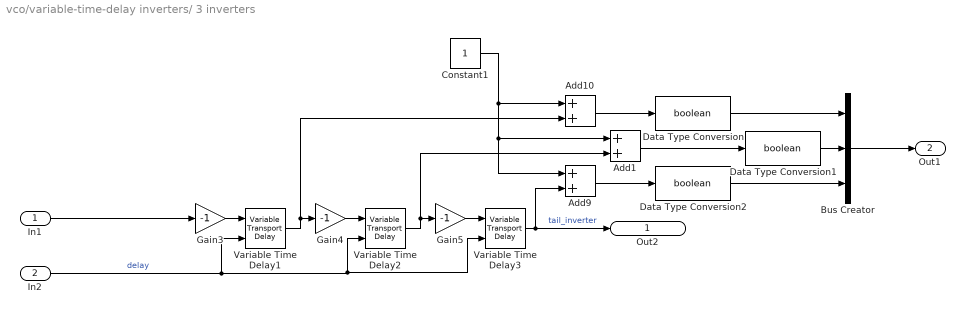
== system vco/variable-time-delay inverters/ 3 inverters ==
  In1 : Inport
  In2 : Inport  Port=2
  Add1 : Sum
  Add10 : Sum
  Add9 : Sum
  Bus Creator : BusCreator  Inputs=3
  Constant1 : Constant  SampleTime=1e-11
  Data Type Conversion : DataTypeConversion  OutDataTypeStr=boolean
  Data Type Conversion1 : DataTypeConversion  OutDataTypeStr=boolean
  Data Type Conversion2 : DataTypeConversion  OutDataTypeStr=boolean
  Gain3 : Gain  Gain=-1
  Gain4 : Gain  Gain=-1
  Gain5 : Gain  Gain=-1
  Variable Time Delay1 : VariableTransportDelay  MaximumDelay=10  InitialOutput=-1
  Variable Time Delay2 : VariableTransportDelay  MaximumDelay=10  InitialOutput=1
  Variable Time Delay3 : VariableTransportDelay  MaximumDelay=10  InitialOutput=-1
  Out2 : Outport
  Out1 : Outport  Port=2
  wires:
  Gain3/1 -> Variable Time Delay1/1
  Gain5/1 -> Variable Time Delay3/1
  Variable Time Delay2/1 -> Add1/2, Gain5/1
  In2/1 -> Variable Time Delay1/2, Variable Time Delay2/2, Variable Time Delay3/2  "delay"
  Gain4/1 -> Variable Time Delay2/1
  Variable Time Delay1/1 -> Add10/2, Gain4/1
  In1/1 -> Gain3/1
  Variable Time Delay3/1 -> Out2/1, Add9/2  "tail_inverter"
  Bus Creator/1 -> Out1/1
  Add9/1 -> Data Type Conversion2/1
  Add1/1 -> Data Type Conversion1/1
  Add10/1 -> Data Type Conversion/1
  Constant1/1 -> Add9/1, Add1/1, Add10/1
  Data Type Conversion2/1 -> Bus Creator/3
  Data Type Conversion1/1 -> Bus Creator/2
  Data Type Conversion/1 -> Bus Creator/1

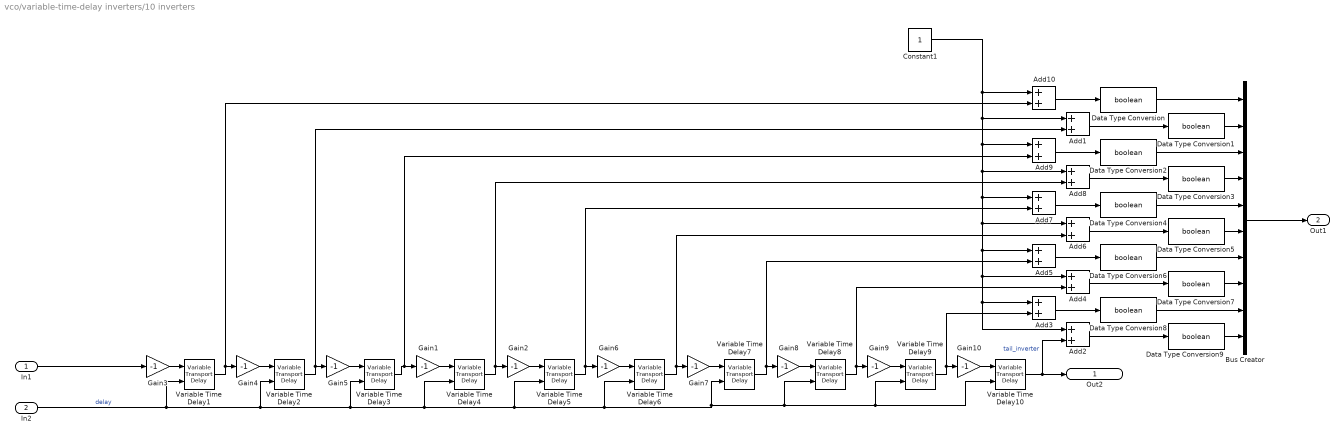
== system vco/variable-time-delay inverters/10 inverters ==
  In1 : Inport
  In2 : Inport  Port=2
  Add{1..10} (10 alike) : Sum
  Bus Creator : BusCreator  Inputs=10
  Constant1 : Constant  SampleTime=1e-11
  Data Type Conversion{,1..9} (10 alike) : DataTypeConversion  OutDataTypeStr=boolean
  Gain{1..10} (10 alike) : Gain  Gain=-1
  Variable Time Delay{1,3,5,7,9} (5 alike) : VariableTransportDelay  MaximumDelay=10  InitialOutput=-1
  Variable Time Delay{2,4,6,8,10} (5 alike) : VariableTransportDelay  MaximumDelay=10  InitialOutput=1
  Out2 : Outport
  Out1 : Outport  Port=2
  wires:
  Gain3/1 -> Variable Time Delay1/1
  Gain5/1 -> Variable Time Delay3/1
  Variable Time Delay6/1 -> Add6/2, Gain7/1
  Variable Time Delay7/1 -> Add5/2, Gain8/1
  Variable Time Delay8/1 -> Add4/2, Gain9/1
  Gain9/1 -> Variable Time Delay9/1
  Variable Time Delay3/1 -> Add9/2, Gain1/1
  Variable Time Delay2/1 -> Add1/2, Gain5/1
  In2/1 -> Variable Time Delay1/2, Variable Time Delay2/2, Variable Time Delay10/2, Variable Time Delay9/2, Variable Time Delay8/2, Variable Time Delay7/2, Variable Time Delay6/2, Variable Time Delay5/2, Variable Time Delay4/2, Variable Time Delay3/2  "delay"
  Gain4/1 -> Variable Time Delay2/1
  Gain10/1 -> Variable Time Delay10/1
  Gain8/1 -> Variable Time Delay8/1
  Variable Time Delay1/1 -> Add10/2, Gain4/1
  Variable Time Delay4/1 -> Add8/2, Gain2/1
  Gain2/1 -> Variable Time Delay5/1
  Gain7/1 -> Variable Time Delay7/1
  Variable Time Delay5/1 -> Add7/2, Gain6/1
  Variable Time Delay9/1 -> Add3/2, Gain10/1
  Gain6/1 -> Variable Time Delay6/1
  Gain1/1 -> Variable Time Delay4/1
  In1/1 -> Gain3/1
  Variable Time Delay10/1 -> Add2/2, Out2/1  "tail_inverter"
  Bus Creator/1 -> Out1/1
  Add2/1 -> Data Type Conversion9/1
  Add3/1 -> Data Type Conversion8/1
  Add5/1 -> Data Type Conversion6/1
  Add4/1 -> Data Type Conversion7/1
  Add6/1 -> Data Type Conversion5/1
  Add9/1 -> Data Type Conversion2/1
  Add7/1 -> Data Type Conversion4/1
  Add8/1 -> Data Type Conversion3/1
  Add1/1 -> Data Type Conversion1/1
  Add10/1 -> Data Type Conversion/1
  Constant1/1 -> Add2/1, Add3/1, Add4/1, Add5/1, Add6/1, Add7/1, Add8/1, Add9/1, Add1/1, Add10/1
  Data Type Conversion/1 -> Bus Creator/1
  Data Type Conversion1/1 -> Bus Creator/2
  Data Type Conversion3/1 -> Bus Creator/4
  Data Type Conversion2/1 -> Bus Creator/3
  Data Type Conversion4/1 -> Bus Creator/5
  Data Type Conversion5/1 -> Bus Creator/6
  Data Type Conversion6/1 -> Bus Creator/7
  Data Type Conversion7/1 -> Bus Creator/8
  Data Type Conversion8/1 -> Bus Creator/9
  Data Type Conversion9/1 -> Bus Creator/10

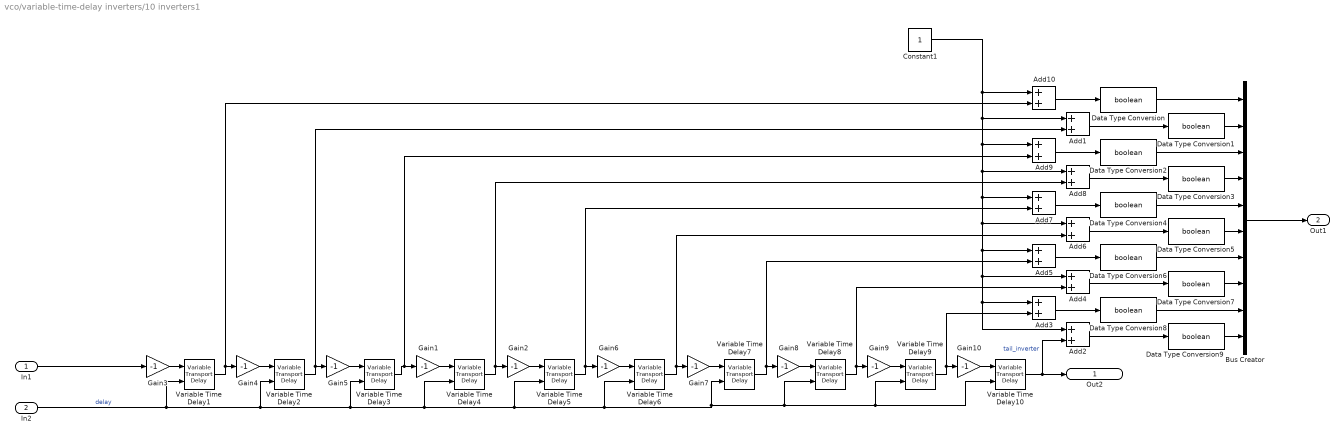
== system vco/variable-time-delay inverters/10 inverters1 ==
  In1 : Inport
  In2 : Inport  Port=2
  Add{1..10} (10 alike) : Sum
  Bus Creator : BusCreator  Inputs=10
  Constant1 : Constant  SampleTime=1e-11
  Data Type Conversion{,1..9} (10 alike) : DataTypeConversion  OutDataTypeStr=boolean
  Gain{1..10} (10 alike) : Gain  Gain=-1
  Variable Time Delay{1,3,5,7,9} (5 alike) : VariableTransportDelay  MaximumDelay=10  InitialOutput=-1
  Variable Time Delay{2,4,6,8,10} (5 alike) : VariableTransportDelay  MaximumDelay=10  InitialOutput=1
  Out2 : Outport
  Out1 : Outport  Port=2
  wires:
  Gain3/1 -> Variable Time Delay1/1
  Gain5/1 -> Variable Time Delay3/1
  Variable Time Delay6/1 -> Add6/2, Gain7/1
  Variable Time Delay7/1 -> Add5/2, Gain8/1
  Variable Time Delay8/1 -> Add4/2, Gain9/1
  Gain9/1 -> Variable Time Delay9/1
  Variable Time Delay3/1 -> Add9/2, Gain1/1
  Variable Time Delay2/1 -> Add1/2, Gain5/1
  In2/1 -> Variable Time Delay1/2, Variable Time Delay2/2, Variable Time Delay10/2, Variable Time Delay9/2, Variable Time Delay8/2, Variable Time Delay7/2, Variable Time Delay6/2, Variable Time Delay5/2, Variable Time Delay4/2, Variable Time Delay3/2  "delay"
  Gain4/1 -> Variable Time Delay2/1
  Gain10/1 -> Variable Time Delay10/1
  Gain8/1 -> Variable Time Delay8/1
  Variable Time Delay1/1 -> Add10/2, Gain4/1
  Variable Time Delay4/1 -> Add8/2, Gain2/1
  Gain2/1 -> Variable Time Delay5/1
  Gain7/1 -> Variable Time Delay7/1
  Variable Time Delay5/1 -> Add7/2, Gain6/1
  Variable Time Delay9/1 -> Add3/2, Gain10/1
  Gain6/1 -> Variable Time Delay6/1
  Gain1/1 -> Variable Time Delay4/1
  In1/1 -> Gain3/1
  Variable Time Delay10/1 -> Add2/2, Out2/1  "tail_inverter"
  Bus Creator/1 -> Out1/1
  Add2/1 -> Data Type Conversion9/1
  Add3/1 -> Data Type Conversion8/1
  Add5/1 -> Data Type Conversion6/1
  Add4/1 -> Data Type Conversion7/1
  Add6/1 -> Data Type Conversion5/1
  Add9/1 -> Data Type Conversion2/1
  Add7/1 -> Data Type Conversion4/1
  Add8/1 -> Data Type Conversion3/1
  Add1/1 -> Data Type Conversion1/1
  Add10/1 -> Data Type Conversion/1
  Constant1/1 -> Add2/1, Add3/1, Add4/1, Add5/1, Add6/1, Add7/1, Add8/1, Add9/1, Add1/1, Add10/1
  Data Type Conversion/1 -> Bus Creator/1
  Data Type Conversion1/1 -> Bus Creator/2
  Data Type Conversion3/1 -> Bus Creator/4
  Data Type Conversion2/1 -> Bus Creator/3
  Data Type Conversion4/1 -> Bus Creator/5
  Data Type Conversion5/1 -> Bus Creator/6
  Data Type Conversion6/1 -> Bus Creator/7
  Data Type Conversion7/1 -> Bus Creator/8
  Data Type Conversion8/1 -> Bus Creator/9
  Data Type Conversion9/1 -> Bus Creator/10

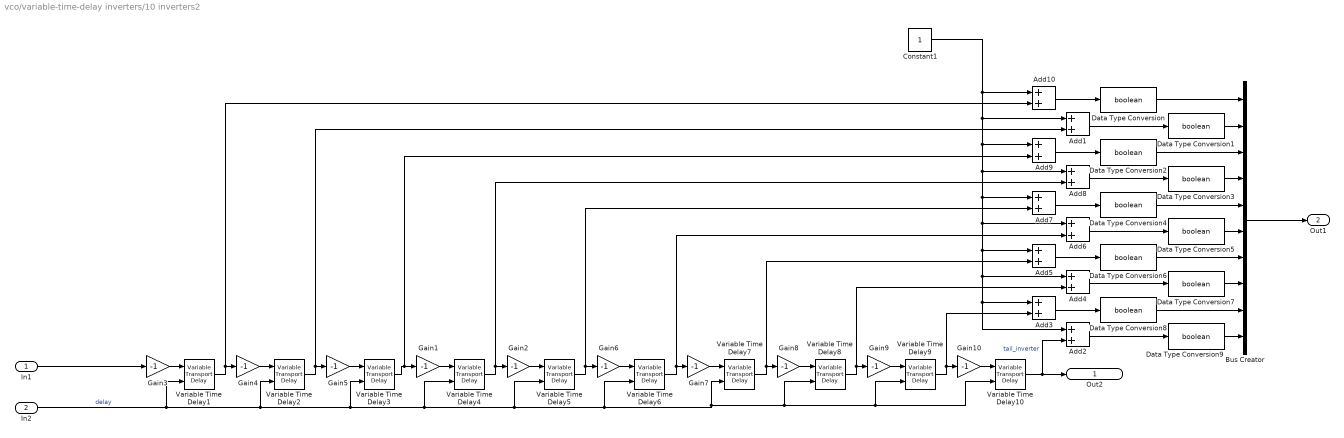
== system vco/variable-time-delay inverters/10 inverters2 ==
  In1 : Inport
  In2 : Inport  Port=2
  Add{1..10} (10 alike) : Sum
  Bus Creator : BusCreator  Inputs=10
  Constant1 : Constant  SampleTime=1e-11
  Data Type Conversion{,1..9} (10 alike) : DataTypeConversion  OutDataTypeStr=boolean
  Gain{1..10} (10 alike) : Gain  Gain=-1
  Variable Time Delay{1,3,5,7,9} (5 alike) : VariableTransportDelay  MaximumDelay=10  InitialOutput=-1
  Variable Time Delay{2,4,6,8,10} (5 alike) : VariableTransportDelay  MaximumDelay=10  InitialOutput=1
  Out2 : Outport
  Out1 : Outport  Port=2
  wires:
  Gain3/1 -> Variable Time Delay1/1
  Gain5/1 -> Variable Time Delay3/1
  Variable Time Delay6/1 -> Add6/2, Gain7/1
  Variable Time Delay7/1 -> Add5/2, Gain8/1
  Variable Time Delay8/1 -> Add4/2, Gain9/1
  Gain9/1 -> Variable Time Delay9/1
  Variable Time Delay3/1 -> Add9/2, Gain1/1
  Variable Time Delay2/1 -> Add1/2, Gain5/1
  In2/1 -> Variable Time Delay1/2, Variable Time Delay2/2, Variable Time Delay10/2, Variable Time Delay9/2, Variable Time Delay8/2, Variable Time Delay7/2, Variable Time Delay6/2, Variable Time Delay5/2, Variable Time Delay4/2, Variable Time Delay3/2  "delay"
  Gain4/1 -> Variable Time Delay2/1
  Gain10/1 -> Variable Time Delay10/1
  Gain8/1 -> Variable Time Delay8/1
  Variable Time Delay1/1 -> Add10/2, Gain4/1
  Variable Time Delay4/1 -> Add8/2, Gain2/1
  Gain2/1 -> Variable Time Delay5/1
  Gain7/1 -> Variable Time Delay7/1
  Variable Time Delay5/1 -> Add7/2, Gain6/1
  Variable Time Delay9/1 -> Add3/2, Gain10/1
  Gain6/1 -> Variable Time Delay6/1
  Gain1/1 -> Variable Time Delay4/1
  In1/1 -> Gain3/1
  Variable Time Delay10/1 -> Add2/2, Out2/1  "tail_inverter"
  Bus Creator/1 -> Out1/1
  Add2/1 -> Data Type Conversion9/1
  Add3/1 -> Data Type Conversion8/1
  Add5/1 -> Data Type Conversion6/1
  Add4/1 -> Data Type Conversion7/1
  Add6/1 -> Data Type Conversion5/1
  Add9/1 -> Data Type Conversion2/1
  Add7/1 -> Data Type Conversion4/1
  Add8/1 -> Data Type Conversion3/1
  Add1/1 -> Data Type Conversion1/1
  Add10/1 -> Data Type Conversion/1
  Constant1/1 -> Add2/1, Add3/1, Add4/1, Add5/1, Add6/1, Add7/1, Add8/1, Add9/1, Add1/1, Add10/1
  Data Type Conversion/1 -> Bus Creator/1
  Data Type Conversion1/1 -> Bus Creator/2
  Data Type Conversion3/1 -> Bus Creator/4
  Data Type Conversion2/1 -> Bus Creator/3
  Data Type Conversion4/1 -> Bus Creator/5
  Data Type Conversion5/1 -> Bus Creator/6
  Data Type Conversion6/1 -> Bus Creator/7
  Data Type Conversion7/1 -> Bus Creator/8
  Data Type Conversion8/1 -> Bus Creator/9
  Data Type Conversion9/1 -> Bus Creator/10

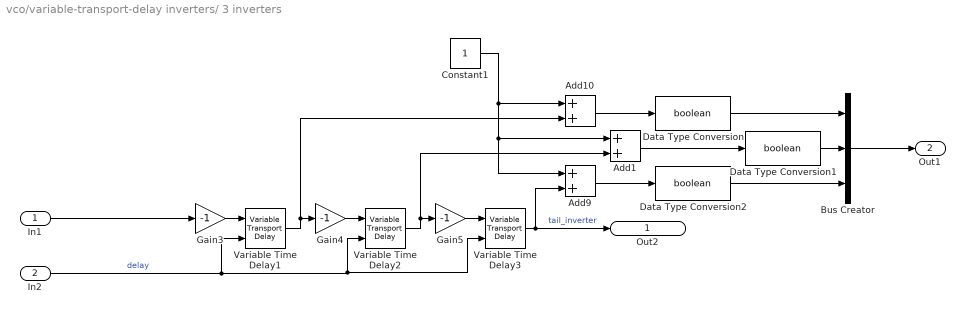
== system vco/variable-transport-delay inverters/ 3 inverters ==
  In1 : Inport
  In2 : Inport  Port=2
  Add1 : Sum
  Add10 : Sum
  Add9 : Sum
  Bus Creator : BusCreator  Inputs=3
  Constant1 : Constant  SampleTime=1e-11
  Data Type Conversion : DataTypeConversion  OutDataTypeStr=boolean
  Data Type Conversion1 : DataTypeConversion  OutDataTypeStr=boolean
  Data Type Conversion2 : DataTypeConversion  OutDataTypeStr=boolean
  Gain3 : Gain  Gain=-1
  Gain4 : Gain  Gain=-1
  Gain5 : Gain  Gain=-1
  Variable Time Delay1 : VariableTransportDelay  VariableDelayType=Variable transport delay  MaximumDelay=10  InitialOutput=-1
  Variable Time Delay2 : VariableTransportDelay  VariableDelayType=Variable transport delay  MaximumDelay=10  InitialOutput=1
  Variable Time Delay3 : VariableTransportDelay  VariableDelayType=Variable transport delay  MaximumDelay=10  InitialOutput=-1
  Out2 : Outport
  Out1 : Outport  Port=2
  wires:
  Gain3/1 -> Variable Time Delay1/1
  Gain5/1 -> Variable Time Delay3/1
  Variable Time Delay2/1 -> Add1/2, Gain5/1
  In2/1 -> Variable Time Delay1/2, Variable Time Delay2/2, Variable Time Delay3/2  "delay"
  Gain4/1 -> Variable Time Delay2/1
  Variable Time Delay1/1 -> Add10/2, Gain4/1
  In1/1 -> Gain3/1
  Variable Time Delay3/1 -> Out2/1, Add9/2  "tail_inverter"
  Bus Creator/1 -> Out1/1
  Add9/1 -> Data Type Conversion2/1
  Add1/1 -> Data Type Conversion1/1
  Add10/1 -> Data Type Conversion/1
  Constant1/1 -> Add9/1, Add1/1, Add10/1
  Data Type Conversion2/1 -> Bus Creator/3
  Data Type Conversion1/1 -> Bus Creator/2
  Data Type Conversion/1 -> Bus Creator/1

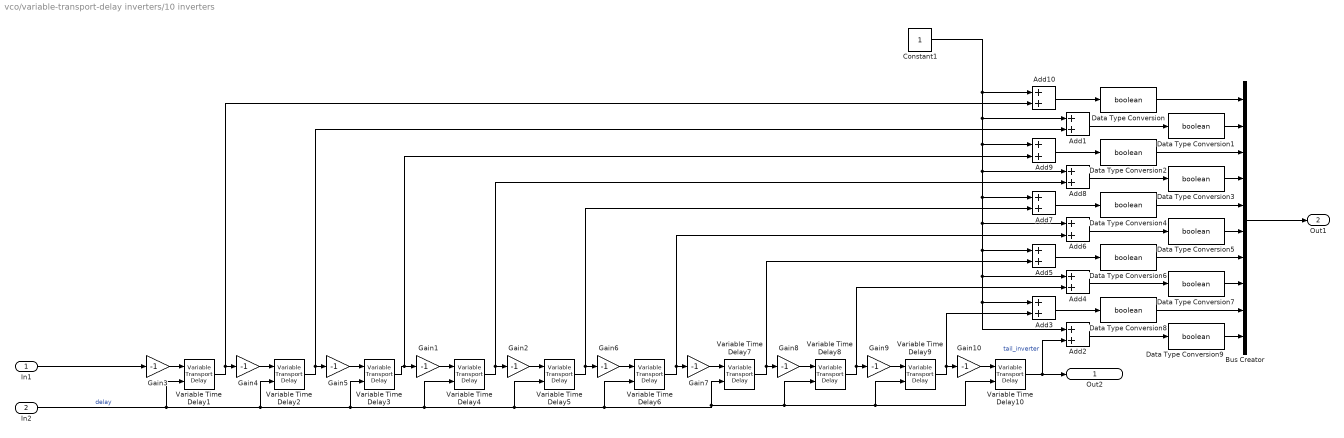
== system vco/variable-transport-delay inverters/10 inverters ==
  In1 : Inport
  In2 : Inport  Port=2
  Add{1..10} (10 alike) : Sum
  Bus Creator : BusCreator  Inputs=10
  Constant1 : Constant  SampleTime=1e-11
  Data Type Conversion{,1..9} (10 alike) : DataTypeConversion  OutDataTypeStr=boolean
  Gain{1..10} (10 alike) : Gain  Gain=-1
  Variable Time Delay{1,3,5,7,9} (5 alike) : VariableTransportDelay  VariableDelayType=Variable transport delay  MaximumDelay=10  InitialOutput=-1
  Variable Time Delay{2,4,6,8,10} (5 alike) : VariableTransportDelay  VariableDelayType=Variable transport delay  MaximumDelay=10  InitialOutput=1
  Out2 : Outport
  Out1 : Outport  Port=2
  wires:
  Gain3/1 -> Variable Time Delay1/1
  Gain5/1 -> Variable Time Delay3/1
  Variable Time Delay6/1 -> Add6/2, Gain7/1
  Variable Time Delay7/1 -> Add5/2, Gain8/1
  Variable Time Delay8/1 -> Add4/2, Gain9/1
  Gain9/1 -> Variable Time Delay9/1
  Variable Time Delay3/1 -> Add9/2, Gain1/1
  Variable Time Delay2/1 -> Add1/2, Gain5/1
  In2/1 -> Variable Time Delay1/2, Variable Time Delay2/2, Variable Time Delay10/2, Variable Time Delay9/2, Variable Time Delay8/2, Variable Time Delay7/2, Variable Time Delay6/2, Variable Time Delay5/2, Variable Time Delay4/2, Variable Time Delay3/2  "delay"
  Gain4/1 -> Variable Time Delay2/1
  Gain10/1 -> Variable Time Delay10/1
  Gain8/1 -> Variable Time Delay8/1
  Variable Time Delay1/1 -> Add10/2, Gain4/1
  Variable Time Delay4/1 -> Add8/2, Gain2/1
  Gain2/1 -> Variable Time Delay5/1
  Gain7/1 -> Variable Time Delay7/1
  Variable Time Delay5/1 -> Add7/2, Gain6/1
  Variable Time Delay9/1 -> Add3/2, Gain10/1
  Gain6/1 -> Variable Time Delay6/1
  Gain1/1 -> Variable Time Delay4/1
  In1/1 -> Gain3/1
  Variable Time Delay10/1 -> Add2/2, Out2/1  "tail_inverter"
  Bus Creator/1 -> Out1/1
  Add2/1 -> Data Type Conversion9/1
  Add3/1 -> Data Type Conversion8/1
  Add5/1 -> Data Type Conversion6/1
  Add4/1 -> Data Type Conversion7/1
  Add6/1 -> Data Type Conversion5/1
  Add9/1 -> Data Type Conversion2/1
  Add7/1 -> Data Type Conversion4/1
  Add8/1 -> Data Type Conversion3/1
  Add1/1 -> Data Type Conversion1/1
  Add10/1 -> Data Type Conversion/1
  Constant1/1 -> Add2/1, Add3/1, Add4/1, Add5/1, Add6/1, Add7/1, Add8/1, Add9/1, Add1/1, Add10/1
  Data Type Conversion/1 -> Bus Creator/1
  Data Type Conversion1/1 -> Bus Creator/2
  Data Type Conversion3/1 -> Bus Creator/4
  Data Type Conversion2/1 -> Bus Creator/3
  Data Type Conversion4/1 -> Bus Creator/5
  Data Type Conversion5/1 -> Bus Creator/6
  Data Type Conversion6/1 -> Bus Creator/7
  Data Type Conversion7/1 -> Bus Creator/8
  Data Type Conversion8/1 -> Bus Creator/9
  Data Type Conversion9/1 -> Bus Creator/10

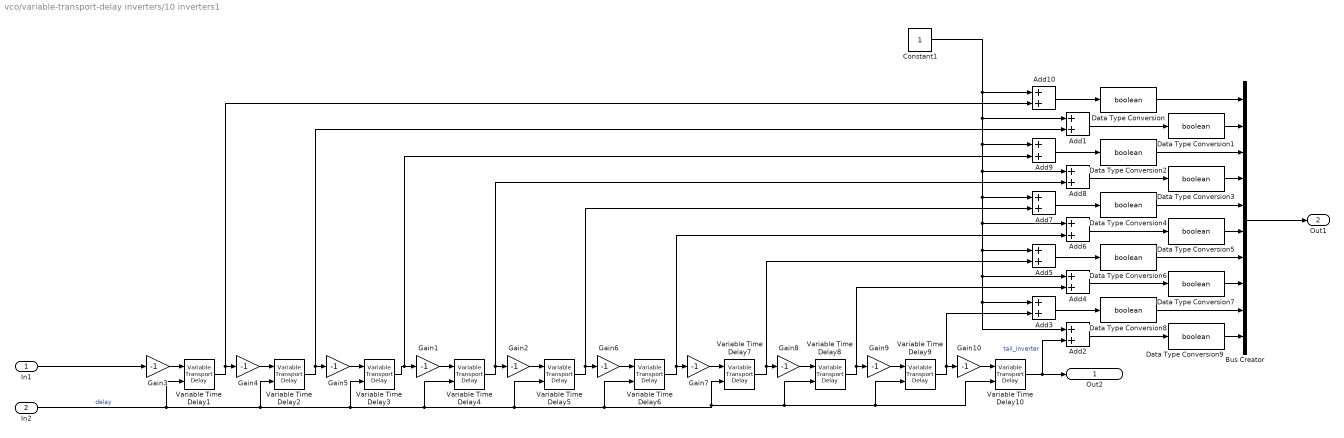
== system vco/variable-transport-delay inverters/10 inverters1 ==
  In1 : Inport
  In2 : Inport  Port=2
  Add{1..10} (10 alike) : Sum
  Bus Creator : BusCreator  Inputs=10
  Constant1 : Constant  SampleTime=1e-11
  Data Type Conversion{,1..9} (10 alike) : DataTypeConversion  OutDataTypeStr=boolean
  Gain{1..10} (10 alike) : Gain  Gain=-1
  Variable Time Delay{1,3,5,7,9} (5 alike) : VariableTransportDelay  VariableDelayType=Variable transport delay  MaximumDelay=10  InitialOutput=-1
  Variable Time Delay{2,4,6,8,10} (5 alike) : VariableTransportDelay  VariableDelayType=Variable transport delay  MaximumDelay=10  InitialOutput=1
  Out2 : Outport
  Out1 : Outport  Port=2
  wires:
  Gain3/1 -> Variable Time Delay1/1
  Gain5/1 -> Variable Time Delay3/1
  Variable Time Delay6/1 -> Add6/2, Gain7/1
  Variable Time Delay7/1 -> Add5/2, Gain8/1
  Variable Time Delay8/1 -> Add4/2, Gain9/1
  Gain9/1 -> Variable Time Delay9/1
  Variable Time Delay3/1 -> Add9/2, Gain1/1
  Variable Time Delay2/1 -> Add1/2, Gain5/1
  In2/1 -> Variable Time Delay1/2, Variable Time Delay2/2, Variable Time Delay10/2, Variable Time Delay9/2, Variable Time Delay8/2, Variable Time Delay7/2, Variable Time Delay6/2, Variable Time Delay5/2, Variable Time Delay4/2, Variable Time Delay3/2  "delay"
  Gain4/1 -> Variable Time Delay2/1
  Gain10/1 -> Variable Time Delay10/1
  Gain8/1 -> Variable Time Delay8/1
  Variable Time Delay1/1 -> Add10/2, Gain4/1
  Variable Time Delay4/1 -> Add8/2, Gain2/1
  Gain2/1 -> Variable Time Delay5/1
  Gain7/1 -> Variable Time Delay7/1
  Variable Time Delay5/1 -> Add7/2, Gain6/1
  Variable Time Delay9/1 -> Add3/2, Gain10/1
  Gain6/1 -> Variable Time Delay6/1
  Gain1/1 -> Variable Time Delay4/1
  In1/1 -> Gain3/1
  Variable Time Delay10/1 -> Add2/2, Out2/1  "tail_inverter"
  Bus Creator/1 -> Out1/1
  Add2/1 -> Data Type Conversion9/1
  Add3/1 -> Data Type Conversion8/1
  Add5/1 -> Data Type Conversion6/1
  Add4/1 -> Data Type Conversion7/1
  Add6/1 -> Data Type Conversion5/1
  Add9/1 -> Data Type Conversion2/1
  Add7/1 -> Data Type Conversion4/1
  Add8/1 -> Data Type Conversion3/1
  Add1/1 -> Data Type Conversion1/1
  Add10/1 -> Data Type Conversion/1
  Constant1/1 -> Add2/1, Add3/1, Add4/1, Add5/1, Add6/1, Add7/1, Add8/1, Add9/1, Add1/1, Add10/1
  Data Type Conversion/1 -> Bus Creator/1
  Data Type Conversion1/1 -> Bus Creator/2
  Data Type Conversion3/1 -> Bus Creator/4
  Data Type Conversion2/1 -> Bus Creator/3
  Data Type Conversion4/1 -> Bus Creator/5
  Data Type Conversion5/1 -> Bus Creator/6
  Data Type Conversion6/1 -> Bus Creator/7
  Data Type Conversion7/1 -> Bus Creator/8
  Data Type Conversion8/1 -> Bus Creator/9
  Data Type Conversion9/1 -> Bus Creator/10

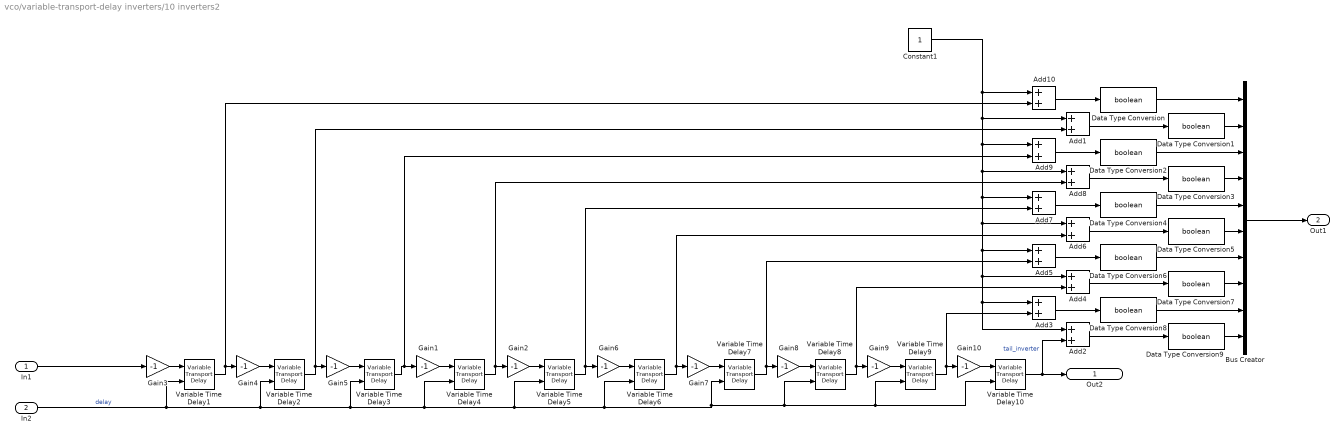
== system vco/variable-transport-delay inverters/10 inverters2 ==
  In1 : Inport
  In2 : Inport  Port=2
  Add{1..10} (10 alike) : Sum
  Bus Creator : BusCreator  Inputs=10
  Constant1 : Constant  SampleTime=1e-11
  Data Type Conversion{,1..9} (10 alike) : DataTypeConversion  OutDataTypeStr=boolean
  Gain{1..10} (10 alike) : Gain  Gain=-1
  Variable Time Delay{1,3,5,7,9} (5 alike) : VariableTransportDelay  VariableDelayType=Variable transport delay  MaximumDelay=10  InitialOutput=-1
  Variable Time Delay{2,4,6,8,10} (5 alike) : VariableTransportDelay  VariableDelayType=Variable transport delay  MaximumDelay=10  InitialOutput=1
  Out2 : Outport
  Out1 : Outport  Port=2
  wires:
  Gain3/1 -> Variable Time Delay1/1
  Gain5/1 -> Variable Time Delay3/1
  Variable Time Delay6/1 -> Add6/2, Gain7/1
  Variable Time Delay7/1 -> Add5/2, Gain8/1
  Variable Time Delay8/1 -> Add4/2, Gain9/1
  Gain9/1 -> Variable Time Delay9/1
  Variable Time Delay3/1 -> Add9/2, Gain1/1
  Variable Time Delay2/1 -> Add1/2, Gain5/1
  In2/1 -> Variable Time Delay1/2, Variable Time Delay2/2, Variable Time Delay10/2, Variable Time Delay9/2, Variable Time Delay8/2, Variable Time Delay7/2, Variable Time Delay6/2, Variable Time Delay5/2, Variable Time Delay4/2, Variable Time Delay3/2  "delay"
  Gain4/1 -> Variable Time Delay2/1
  Gain10/1 -> Variable Time Delay10/1
  Gain8/1 -> Variable Time Delay8/1
  Variable Time Delay1/1 -> Add10/2, Gain4/1
  Variable Time Delay4/1 -> Add8/2, Gain2/1
  Gain2/1 -> Variable Time Delay5/1
  Gain7/1 -> Variable Time Delay7/1
  Variable Time Delay5/1 -> Add7/2, Gain6/1
  Variable Time Delay9/1 -> Add3/2, Gain10/1
  Gain6/1 -> Variable Time Delay6/1
  Gain1/1 -> Variable Time Delay4/1
  In1/1 -> Gain3/1
  Variable Time Delay10/1 -> Add2/2, Out2/1  "tail_inverter"
  Bus Creator/1 -> Out1/1
  Add2/1 -> Data Type Conversion9/1
  Add3/1 -> Data Type Conversion8/1
  Add5/1 -> Data Type Conversion6/1
  Add4/1 -> Data Type Conversion7/1
  Add6/1 -> Data Type Conversion5/1
  Add9/1 -> Data Type Conversion2/1
  Add7/1 -> Data Type Conversion4/1
  Add8/1 -> Data Type Conversion3/1
  Add1/1 -> Data Type Conversion1/1
  Add10/1 -> Data Type Conversion/1
  Constant1/1 -> Add2/1, Add3/1, Add4/1, Add5/1, Add6/1, Add7/1, Add8/1, Add9/1, Add1/1, Add10/1
  Data Type Conversion/1 -> Bus Creator/1
  Data Type Conversion1/1 -> Bus Creator/2
  Data Type Conversion3/1 -> Bus Creator/4
  Data Type Conversion2/1 -> Bus Creator/3
  Data Type Conversion4/1 -> Bus Creator/5
  Data Type Conversion5/1 -> Bus Creator/6
  Data Type Conversion6/1 -> Bus Creator/7
  Data Type Conversion7/1 -> Bus Creator/8
  Data Type Conversion8/1 -> Bus Creator/9
  Data Type Conversion9/1 -> Bus Creator/10

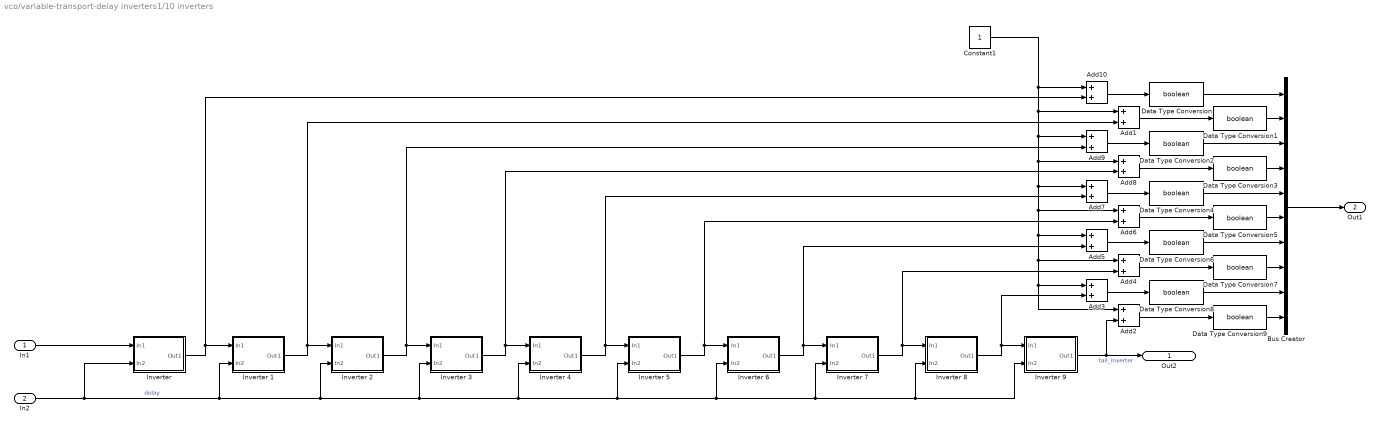
== system vco/variable-transport-delay inverters1/10 inverters ==
  In1 : Inport
  In2 : Inport  Port=2
  Add{1..10} (10 alike) : Sum
  Bus Creator : BusCreator  Inputs=10
  Constant1 : Constant  SampleTime=1e-11
  Data Type Conversion{,1..9} (10 alike) : DataTypeConversion  OutDataTypeStr=boolean
  "Inverter " : Subsystem
  Inverter 1 : Subsystem
  Inverter 2 : Subsystem
  Inverter 3 : Subsystem
  Inverter 4 : Subsystem
  Inverter 5 : Subsystem
  Inverter 6 : Subsystem
  Inverter 7 : Subsystem
  Inverter 8 : Subsystem
  Inverter 9 : Subsystem
  Out2 : Outport
  Out1 : Outport  Port=2
  wires:
  Bus Creator/1 -> Out1/1
  Add2/1 -> Data Type Conversion9/1
  Add3/1 -> Data Type Conversion8/1
  Add5/1 -> Data Type Conversion6/1
  Add4/1 -> Data Type Conversion7/1
  Add6/1 -> Data Type Conversion5/1
  Add9/1 -> Data Type Conversion2/1
  Add7/1 -> Data Type Conversion4/1
  Add8/1 -> Data Type Conversion3/1
  Add1/1 -> Data Type Conversion1/1
  Add10/1 -> Data Type Conversion/1
  Constant1/1 -> Add2/1, Add3/1, Add4/1, Add5/1, Add6/1, Add7/1, Add8/1, Add9/1, Add1/1, Add10/1
  Data Type Conversion/1 -> Bus Creator/1
  Data Type Conversion1/1 -> Bus Creator/2
  Data Type Conversion3/1 -> Bus Creator/4
  Data Type Conversion2/1 -> Bus Creator/3
  Data Type Conversion4/1 -> Bus Creator/5
  Data Type Conversion5/1 -> Bus Creator/6
  Data Type Conversion6/1 -> Bus Creator/7
  Data Type Conversion7/1 -> Bus Creator/8
  Data Type Conversion8/1 -> Bus Creator/9
  Data Type Conversion9/1 -> Bus Creator/10
  "Inverter "/1(Out1) -> Add10/2, Inverter 1/1(In1)
  Inverter 1/1(Out1) -> Add1/2, Inverter 2/1(In1)
  Inverter 2/1(Out1) -> Add9/2, Inverter 3/1(In1)
  Inverter 3/1(Out1) -> Add8/2, Inverter 4/1(In1)
  Inverter 4/1(Out1) -> Add7/2, Inverter 5/1(In1)
  Inverter 5/1(Out1) -> Add6/2, Inverter 6/1(In1)
  Inverter 6/1(Out1) -> Add5/2, Inverter 7/1(In1)
  Inverter 7/1(Out1) -> Add4/2, Inverter 8/1(In1)
  Inverter 8/1(Out1) -> Add3/2, Inverter 9/1(In1)
  In1/1 -> "Inverter "/1(In1)
  In2/1 -> Inverter 9/2(In2), Inverter 8/2(In2), Inverter 7/2(In2), Inverter 6/2(In2), Inverter 5/2(In2), Inverter 4/2(In2), Inverter 3/2(In2), Inverter 2/2(In2), Inverter 1/2(In2), "Inverter "/2(In2)  "delay"
  Inverter 9/1(Out1) -> Add2/2, Out2/1  "tail_inverter"
